simulink model "cycletest_timefeedback"  (R2023a)
settings: Solver=ode1  StartTime=0.0  StopTime=800  FixedStep=0.002  RelTol=1e-3  EnableMultiTasking=on
values from neighbouring files (symbols this model uses):
  cycleGain = 0.2    [simulate_hover.m]    (also in temp.m = 1)
  Jp = 2*Jeq_prop    (= 0.0552224595625)    [setup_lab_hover.m]    (also in simulate_hover.m)
  Jr = 2*Jeq_prop    (= 0.0552224595625)    [setup_lab_hover.m]    (also in simulate_hover.m)
  Jy = 4*Jeq_prop    (= 0.110444919125)    [setup_lab_hover.m]    (also in simulate_hover.m)
  kd = 0.5    [simulate_hover.m]
  Kf = 0.1188    [setup_lab_hover.m]    (also in simulate_hover.m)
  Kt = 0.0036    [setup_lab_hover.m]    (also in simulate_hover.m)
  L = 7.75*0.0254    (= 0.19685)    [setup_lab_hover.m]    (also in simulate_hover.m = 0.1969)
  r = flexSize(no)    [phaseComp.m]    (also in simulate_hover.m = 0.5)
  sigma = 0    [simulate_hover.m]
  skew = 2    [simulate_hover.m]
  V_bias = 12    [setup_lab_hover.m]    (also in simulate_hover.m)
  velMax = 100*60*pi/180    (= 104.71975512)    [simulate_hover.m]
  VMAX_AMP = 24    [setup_lab_hover.m]    (also in simulate_hover.m)
  wcf = 2 * pi * 20    (= 125.663706144)    [setup_lab_hover.m]    (also in simulate_hover.m)
  zetaf = 0.6    [setup_lab_hover.m]    (also in simulate_hover.m)
libraries: simulink_extras x4, dspsrcs4 x1
settings Model: ExtModeTrigDuration=10000  Creator=kille  LastModifiedBy=Jacob
settings SolverCC: AlgebraicLoopSolver=TrustRegion  PositivePriorityOrder=on  AutoInsertRateTranBlk=on
settings DataIOCC: ReturnWorkspaceOutputs=off
settings OptimizationCC: LifeSpan=inf
settings DebuggingCC: UnconnectedInputMsg=warning  UnconnectedOutputMsg=warning  UnconnectedLineMsg=warning  ArithmeticOperatorsInVariantConditions=warning
settings ModelReferenceCC: EnableRefExpFcnMdlSchedulingChecks=on
settings SFSimCC: SimUseLocalCustomCode=off  CustomCodeUndefinedFunction=UseInterfaceOnly
settings RTWCC: Description=QUARC Win64 Target  SystemTargetFile=quarc_win64.tlc  TemplateMakefile=quarc_default_tmf  RTWUseLocalCustomCode=off
settings CodeAppCC: StateflowObjectComments=on
settings STFCustomTargetCC: TargetPreCompLibLocation=C:\PROGRA~3\QUARC\lib\2016a\win64\release  UseToolchainInfoCompliant=off  SystemTargetFile=quarc_win64.tlc
settings GRTTargetCC: TargetPreCompLibLocation=C:\PROGRA~3\QUARC\lib\2016a\win64\release  ParMdlRefBuildCompliant=off  CompOptLevelCompliant=off  CombineOutputUpdateFcns=off  MatFileLogging=off  CPPClassGenCompliant=off  GRTInterface=on  UseToolchainInfoCompliant=off  ExtMode=on  ExtModeMexFile=quarc_comm
settings ConfigComp: CovMetricSettings=dswe

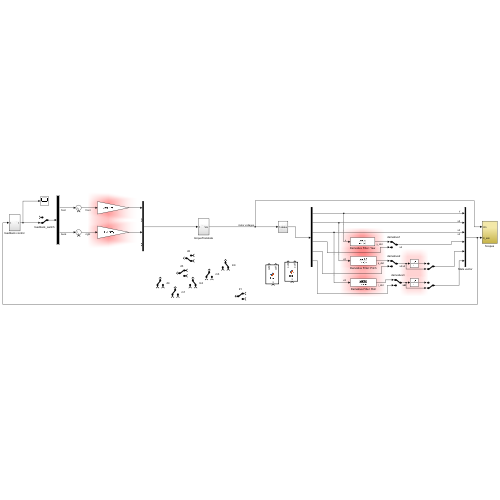
[thumbnail: Simulink's stored preview of the top-level diagram]
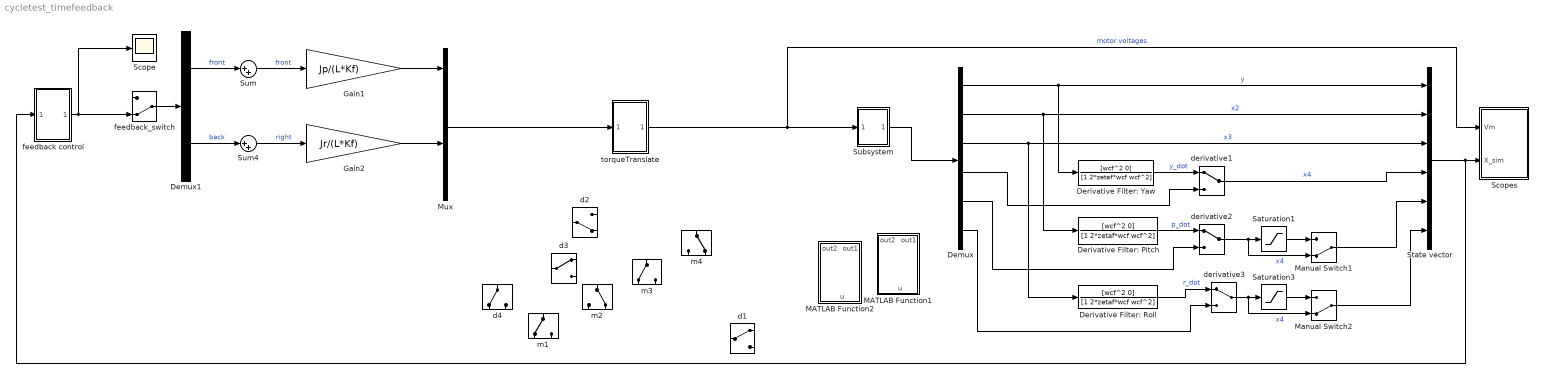
== system cycletest_timefeedback ==
  Demux : Demux  Outputs=6
  Demux1 : Demux  Outputs=2
  Derivative Filter: Pitch : TransferFcn  Numerator=[wcf^2 0]  Denominator=[1 2*zetaf*wcf wcf^2]
  Derivative Filter: Roll : TransferFcn  Numerator=[wcf^2 0]  Denominator=[1 2*zetaf*wcf wcf^2]
  Derivative Filter: Yaw : TransferFcn  Numerator=[wcf^2 0]  Denominator=[1 2*zetaf*wcf wcf^2]
  Gain1 : Gain  Gain=Jp/(L*Kf)
  Gain2 : Gain  Gain=Jr/(L*Kf)
  MATLAB Function1 : MATLAB Function  TreatAsAtomicUnit=on
  MATLAB Function2 : MATLAB Function  TreatAsAtomicUnit=on
  Manual Switch1 : ManualSwitch  CurrentSetting=0
  Manual Switch2 : ManualSwitch  CurrentSetting=0
  Mux : Mux
  Saturation1 : Saturate  UpperLimit=velMax  LowerLimit=-velMax
  Saturation3 : Saturate  UpperLimit=velMax  LowerLimit=-velMax
  Scope : Scope
  Scopes : Subsystem
  State vector : Mux  Inputs=6
  Subsystem : Subsystem
  Sum : Sum  Inputs=|++
  Sum4 : Sum  Inputs=|++
  d1 : ManualSwitch
  d2 : ManualSwitch  CurrentSetting=0
  d3 : ManualSwitch
  d4 : ManualSwitch
  derivative1 : ManualSwitch
  derivative2 : ManualSwitch
  derivative3 : ManualSwitch
  feedback control : Subsystem
  feedback_switch : ManualSwitch  CurrentSetting=0
  m1 : ManualSwitch
  m2 : ManualSwitch  CurrentSetting=0
  m3 : ManualSwitch
  m4 : ManualSwitch  CurrentSetting=0
  torqueTranslate : Subsystem
  wires:
  Demux/1 -> State vector/1, Derivative Filter: Yaw/1  "y"
  torqueTranslate/1(Vm) -> Scopes/1(Vm), Subsystem/1(Input)  "motor voltages"
  Sum4/1 -> Gain2/1  "right"
  Sum/1 -> Gain1/1  "front"
  Mux/1 -> torqueTranslate/1(In1)
  Derivative Filter: Yaw/1 -> derivative1/1  "y_dot"
  Demux/4 -> derivative1/2
  Derivative Filter: Pitch/1 -> derivative2/1  "p_dot"
  Derivative Filter: Roll/1 -> derivative3/1  "r_dot"
  Demux/5 -> derivative2/2
  Demux/6 -> derivative3/2
  derivative1/1 -> State vector/4  "x4"
  derivative2/1 -> Manual Switch1/2, Saturation1/1  "x4"
  Saturation1/1 -> Manual Switch1/1
  derivative3/1 -> Manual Switch2/2, Saturation3/1  "x4"
  Saturation3/1 -> Manual Switch2/1
  Manual Switch1/1 -> State vector/5
  Manual Switch2/1 -> State vector/6
  Demux/3 -> State vector/3, Derivative Filter: Roll/1  "x3"
  Demux/2 -> State vector/2, Derivative Filter: Pitch/1  "x2"
  feedback control/1(Out1) -> Scope/1, feedback_switch/2
  feedback_switch/1 -> Demux1/1
  State vector/1 -> feedback control/1(In1), Scopes/2(X_sim)
  Demux1/1 -> Sum/1  "front"
  Demux1/2 -> Sum4/1  "back"
  Subsystem/1(states) -> Demux/1
  Gain1/1 -> Mux/1
  Gain2/1 -> Mux/3

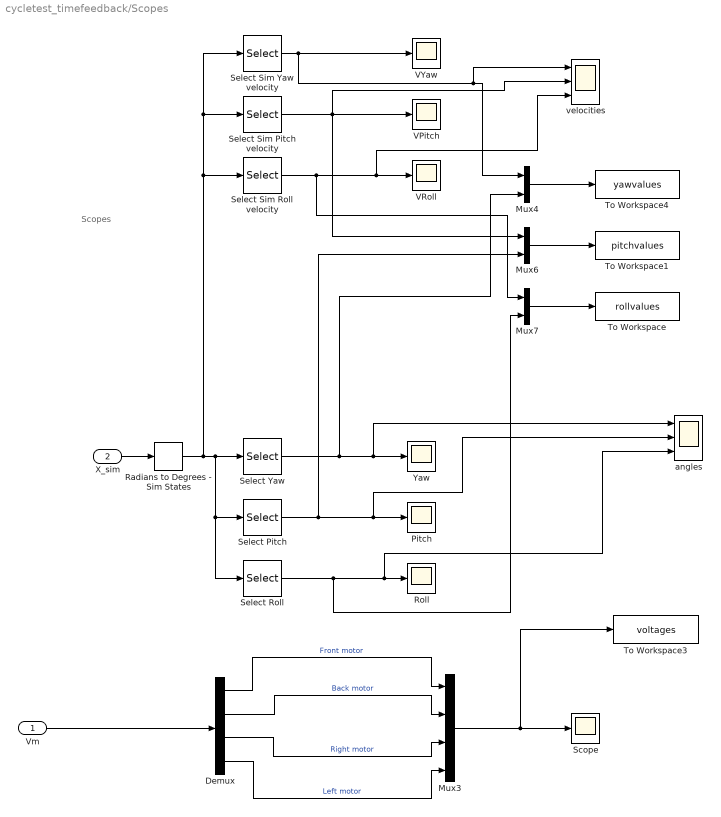
== system cycletest_timefeedback/Scopes ==
  note: Scopes
  Vm : Inport
  X_sim : Inport  Port=2
  Demux : Demux
  Mux3 : Mux
  Mux4 : Mux  Inputs=2
  Mux6 : Mux  Inputs=2
  Mux7 : Mux  Inputs=2
  Pitch : Scope
  Radians to Degrees - Sim States : simulink_extras/Transformations/Radians to Degrees
  Roll : Scope
  Scope : Scope
  Select Pitch : Selector  InputPortWidth=6  IndexOptions=Index vector (dialog)  Indices=2  OutputSizes=1
  Select Roll : Selector  InputPortWidth=6  IndexOptions=Index vector (dialog)  Indices=3  OutputSizes=1
  Select Sim Pitch velocity : Selector  InputPortWidth=6  IndexOptions=Index vector (dialog)  Indices=5  OutputSizes=1
  Select Sim Roll velocity : Selector  InputPortWidth=6  IndexOptions=Index vector (dialog)  Indices=6  OutputSizes=1
  Select Sim Yaw velocity : Selector  InputPortWidth=6  IndexOptions=Index vector (dialog)  Indices=4  OutputSizes=1
  Select Yaw : Selector  InputPortWidth=6  IndexOptions=Index vector (dialog)  Indices=1  OutputSizes=1
  To Workspace : ToWorkspace  VariableName=rollvalues  SampleTime=-1
  To Workspace1 : ToWorkspace  VariableName=pitchvalues  SampleTime=-1
  To Workspace3 : ToWorkspace  VariableName=voltages  SampleTime=-1
  To Workspace4 : ToWorkspace  VariableName=yawvalues  SampleTime=-1
  VPitch : Scope
  VRoll : Scope
  VYaw : Scope
  Yaw : Scope
  angles : Scope  NumInputPorts=3
  velocities : Scope  NumInputPorts=3
  wires:
  Select Roll/1 -> angles/3, Roll/1, Mux7/2
  Radians to Degrees - Sim States/1 -> Select Sim Roll velocity/1, Select Sim Pitch velocity/1, Select Sim Yaw velocity/1, Select Roll/1, Select Pitch/1, Select Yaw/1
  Select Pitch/1 -> angles/2, Pitch/1, Mux6/2
  X_sim/1 -> Radians to Degrees - Sim States/1
  Demux/1 -> Mux3/1  "Front motor"
  Demux/2 -> Mux3/2  "Back motor"
  Demux/3 -> Mux3/3  "Right motor"
  Demux/4 -> Mux3/4  "Left motor"
  Vm/1 -> Demux/1
  Select Sim Yaw velocity/1 -> VYaw/1, velocities/1, Mux4/1
  Select Sim Roll velocity/1 -> velocities/3, VRoll/1, Mux7/1
  Select Sim Pitch velocity/1 -> Mux6/1, velocities/2, VPitch/1
  Mux4/1 -> To Workspace4/1
  Mux6/1 -> To Workspace1/1
  Mux7/1 -> To Workspace/1
  Mux3/1 -> To Workspace3/1, Scope/1
  Select Yaw/1 -> angles/1, Yaw/1, Mux4/2

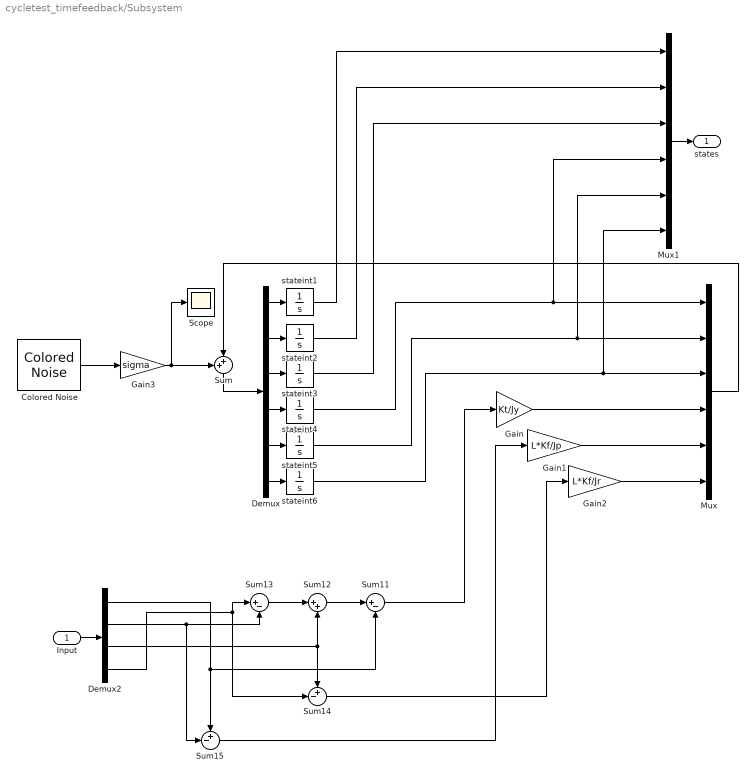
== system cycletest_timefeedback/Subsystem ==
  Input : Inport
  Colored Noise : dspsrcs4/Colored Noise  Color=white  InverseFrequencyPower=1  BoundedOutput=off  NumChannels=6  OutputDataType=double  SamplesPerFrame=1  SampleTime=1  RandomStream=mt19937ar with seed  Seed=67  SimulateUsing=Interpreted execution
  Demux : Demux  Outputs=6
  Demux2 : Demux
  Gain : Gain  Gain=Kt/Jy
  Gain1 : Gain  Gain=L*Kf/Jp
  Gain2 : Gain  Gain=L*Kf/Jr
  Gain3 : Gain  Gain=sigma
  Mux : Mux  Inputs=6
  Mux1 : Mux  Inputs=6
  Scope : Scope
  Sum : Sum  Inputs=++|
  Sum11 : Sum  Inputs=|+-
  Sum12 : Sum  Inputs=|++
  Sum13 : Sum  Inputs=|+-
  Sum14 : Sum  Inputs=+-|
  Sum15 : Sum  Inputs=+-|
  stateint{1,4..6} (4 alike) : Integrator
  stateint2 : Integrator  InitialCondition=0.00010472
  stateint3 : Integrator  InitialCondition=0.00010472
  states : Outport
  wires:
  stateint5/1 -> Mux/2, Mux1/5
  Gain2/1 -> Mux/6
  Gain1/1 -> Mux/5
  stateint6/1 -> Mux/3, Mux1/6
  stateint4/1 -> Mux/1, Mux1/4
  Gain/1 -> Mux/4
  Mux/1 -> Sum/2
  Gain3/1 -> Scope/1, Sum/1
  Demux2/4 -> Sum13/1, Sum14/2
  Demux2/1 -> Sum15/1, Sum11/2
  Demux2/2 -> Sum13/2, Sum15/2
  Sum12/1 -> Sum11/1
  Sum11/1 -> Gain/1
  Demux2/3 -> Sum12/2, Sum14/1
  Sum13/1 -> Sum12/1
  Input/1 -> Demux2/1
  Sum/1 -> Demux/1
  Demux/1 -> stateint1/1
  Demux/2 -> stateint2/1
  Demux/3 -> stateint3/1
  Demux/4 -> stateint4/1
  Demux/5 -> stateint5/1
  Demux/6 -> stateint6/1
  Mux1/1 -> states/1
  stateint1/1 -> Mux1/1
  stateint2/1 -> Mux1/2
  stateint3/1 -> Mux1/3
  Sum15/1 -> Gain1/1
  Sum14/1 -> Gain2/1
  Colored Noise/1 -> Gain3/1

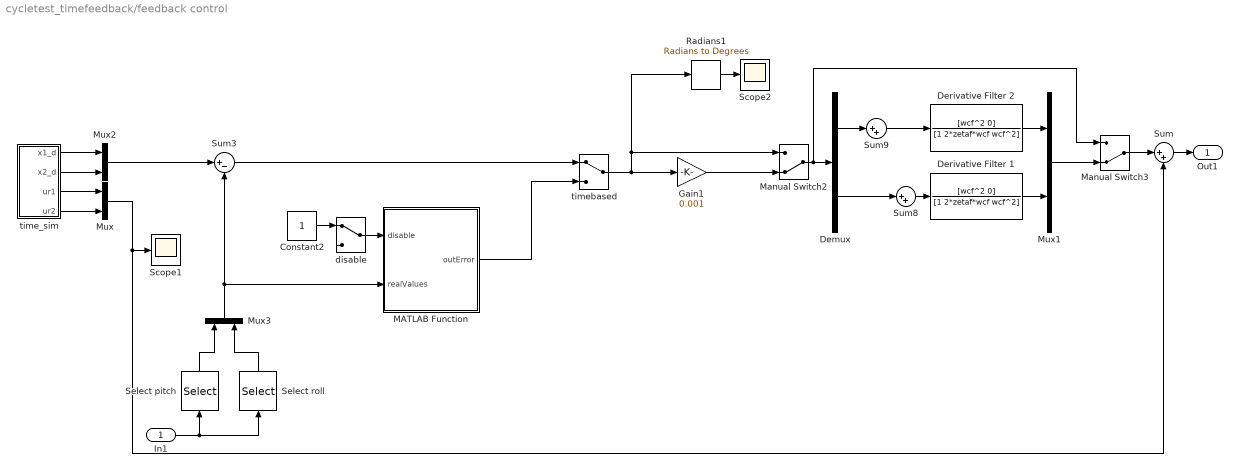
== system cycletest_timefeedback/feedback control ==
  In1 : Inport
  Constant2 : Constant
  Demux : Demux  Outputs=2
  Derivative Filter 1 : TransferFcn  Numerator=[wcf^2 0]  Denominator=[1 2*zetaf*wcf wcf^2]
  Derivative Filter 2 : TransferFcn  Numerator=[wcf^2 0]  Denominator=[1 2*zetaf*wcf wcf^2]
  Gain1 : Gain  Gain=0.001
  MATLAB Function : MATLAB Function  TreatAsAtomicUnit=on
  Manual Switch2 : ManualSwitch  CurrentSetting=0
  Manual Switch3 : ManualSwitch  CurrentSetting=0
  Mux{,1..3} (4 alike) : Mux  Inputs=2
  Radians1 : simulink_extras/Transformations/Radians to Degrees
  Scope1 : Scope
  Scope2 : Scope
  Select pitch : Selector  InputPortWidth=6  IndexOptions=Index vector (dialog)  Indices=2  OutputSizes=1
  Select roll : Selector  InputPortWidth=6  IndexOptions=Index vector (dialog)  Indices=3  OutputSizes=1
  Sum : Sum  Inputs=|++
  Sum3 : Sum  Inputs=|+-
  Sum8 : Sum  Inputs=|++
  Sum9 : Sum  Inputs=|++
  disable : ManualSwitch
  time_sim : Subsystem
  timebased : ManualSwitch
  Out1 : Outport
  wires:
  time_sim/1(x1_d) -> Mux2/1
  time_sim/2(x2_d) -> Mux2/2
  time_sim/4(ur2) -> Mux/2
  time_sim/3(ur1) -> Mux/1
  Sum9/1 -> Derivative Filter 2/1
  Select pitch/1 -> Mux3/1
  Select roll/1 -> Mux3/2
  Sum/1 -> Out1/1
  Sum3/1 -> timebased/1
  Gain1/1 -> Manual Switch2/2
  Mux1/1 -> Manual Switch3/2
  Derivative Filter 2/1 -> Mux1/1
  MATLAB Function/1(outError) -> timebased/2
  Derivative Filter 1/1 -> Mux1/2
  Demux/1 -> Sum9/1
  Mux3/1 -> MATLAB Function/2(realValues), Sum3/2
  Radians1/1 -> Scope2/1
  Manual Switch2/1 -> Manual Switch3/1, Demux/1
  Sum8/1 -> Derivative Filter 1/1
  disable/1 -> MATLAB Function/1(disable)
  In1/1 -> Select roll/1, Select pitch/1
  Mux2/1 -> Sum3/1
  Mux/1 -> Sum/2, Scope1/1
  Constant2/1 -> disable/1
  Demux/2 -> Sum8/1
  Manual Switch3/1 -> Sum/1
  timebased/1 -> Manual Switch2/1, Radians1/1, Gain1/1

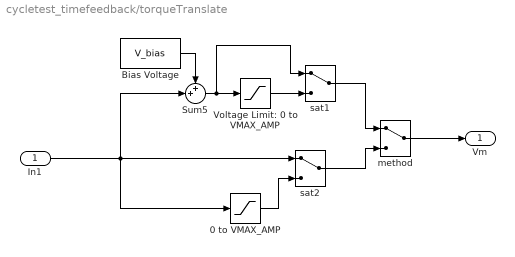
== system cycletest_timefeedback/torqueTranslate ==
  In1 : Inport
  0 to VMAX_AMP : Saturate  UpperLimit=VMAX_AMP  LowerLimit=0
  Bias Voltage : Constant  Value=V_bias
  Sum5 : Sum  Inputs=++|
  Voltage Limit: 0 to VMAX_AMP : Saturate  UpperLimit=VMAX_AMP  LowerLimit=0
  method : ManualSwitch  Tag=swt
  sat1 : ManualSwitch
  sat2 : ManualSwitch
  Vm : Outport
  wires:
  Sum5/1 -> sat1/1, Voltage Limit: 0 to VMAX_AMP/1
  Bias Voltage/1 -> Sum5/1
  Voltage Limit: 0 to VMAX_AMP/1 -> sat1/2
  0 to VMAX_AMP/1 -> sat2/2
  sat1/1 -> method/1
  method/1 -> Vm/1
  sat2/1 -> method/2
  In1/1 -> 0 to VMAX_AMP/1, sat2/1, Sum5/2

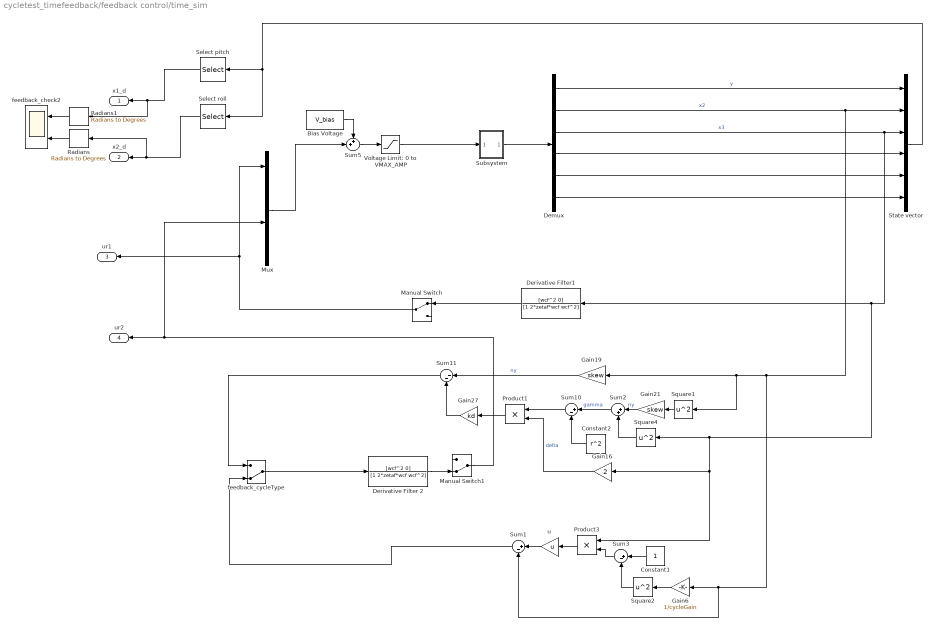
== system cycletest_timefeedback/feedback control/time_sim ==
  Bias Voltage : Constant  Value=V_bias
  Constant1 : Constant
  Constant2 : Constant  Value=r^2
  Demux : Demux  Outputs=6
  Derivative Filter 2 : TransferFcn  Numerator=[wcf^2 0]  Denominator=[1 2*zetaf*wcf wcf^2]
  Derivative Filter1 : TransferFcn  Numerator=[wcf^2 0]  Denominator=[1 2*zetaf*wcf wcf^2]
  Gain16 : Gain  Gain=2
  Gain19 : Gain  Gain=skew
  Gain21 : Gain  Gain=skew
  Gain27 : Gain  Gain=kd
  Gain6 : Gain  Gain=1/cycleGain
  Manual Switch : ManualSwitch
  Manual Switch1 : ManualSwitch  CurrentSetting=0
  Mux : Mux
  Product1 : Product
  Product3 : Product
  Radians : simulink_extras/Transformations/Radians to Degrees
  Radians1 : simulink_extras/Transformations/Radians to Degrees
  Select pitch : Selector  InputPortWidth=6  IndexOptions=Index vector (dialog)  Indices=2  OutputSizes=1
  Select roll : Selector  InputPortWidth=6  IndexOptions=Index vector (dialog)  Indices=3  OutputSizes=1
  Square1 : Math  Operator=square
  Square2 : Math  Operator=square
  Square4 : Math  Operator=square
  State vector : Mux  Inputs=6
  Subsystem : Subsystem
  Sum1 : Sum  Inputs=|+-
  Sum10 : Sum  Inputs=|+-
  Sum11 : Sum  Inputs=|--
  Sum2 : Sum  Inputs=|++
  Sum3 : Sum  Inputs=|+-
  Sum5 : Sum  Inputs=++|
  Voltage Limit: 0 to VMAX_AMP : Saturate  UpperLimit=VMAX_AMP  LowerLimit=0
  feedback_check2 : Scope  NumInputPorts=2
  feedback_cycleType : ManualSwitch  CurrentSetting=0
  u : Gain  Gain=u
  x1_d : Outport
  x2_d : Outport  Port=2
  ur1 : Outport  Port=3
  ur2 : Outport  Port=4
  wires:
  Radians1/1 -> feedback_check2/1
  Radians/1 -> feedback_check2/2
  Bias Voltage/1 -> Sum5/1
  Sum5/1 -> Voltage Limit: 0 to VMAX_AMP/1
  Mux/1 -> Sum5/2
  Select roll/1 -> Radians/1, x2_d/1
  Select pitch/1 -> Radians1/1, x1_d/1
  Demux/4 -> State vector/4
  Demux/6 -> State vector/6
  Subsystem/1(states) -> Demux/1
  Demux/5 -> State vector/5
  Demux/1 -> State vector/1  "y"
  Voltage Limit: 0 to VMAX_AMP/1 -> Subsystem/1(Input)
  State vector/1 -> Select roll/1, Select pitch/1
  Sum1/1 -> feedback_cycleType/2
  Constant1/1 -> Sum3/1
  Gain27/1 -> Sum11/2
  Sum10/1 -> Product1/1
  Product1/1 -> Gain27/1
  feedback_cycleType/1 -> Derivative Filter 2/1
  Derivative Filter 2/1 -> Manual Switch1/2
  Product3/1 -> u/1
  Demux/2 -> State vector/2, Gain6/1, Sum1/2, Square1/1, Gain19/1  "x2"
  Square2/1 -> Sum3/2
  Gain16/1 -> Product1/2  "delta"
  Square1/1 -> Gain21/1
  Sum11/1 -> feedback_cycleType/1
  Sum2/1 -> Sum10/1  "gamma"
  Constant2/1 -> Sum10/2
  Square4/1 -> Sum2/2
  Gain21/1 -> Sum2/1  "ny"
  Derivative Filter1/1 -> Manual Switch/1
  u/1 -> Sum1/1
  Manual Switch1/1 -> Mux/3, ur2/1
  Demux/3 -> Derivative Filter1/1, Product3/1, Gain16/1, Square4/1, State vector/3  "x3"
  Gain19/1 -> Sum11/1  "ny"
  Sum3/1 -> Product3/2
  Manual Switch/1 -> Mux/1, ur1/1
  Gain6/1 -> Square2/1

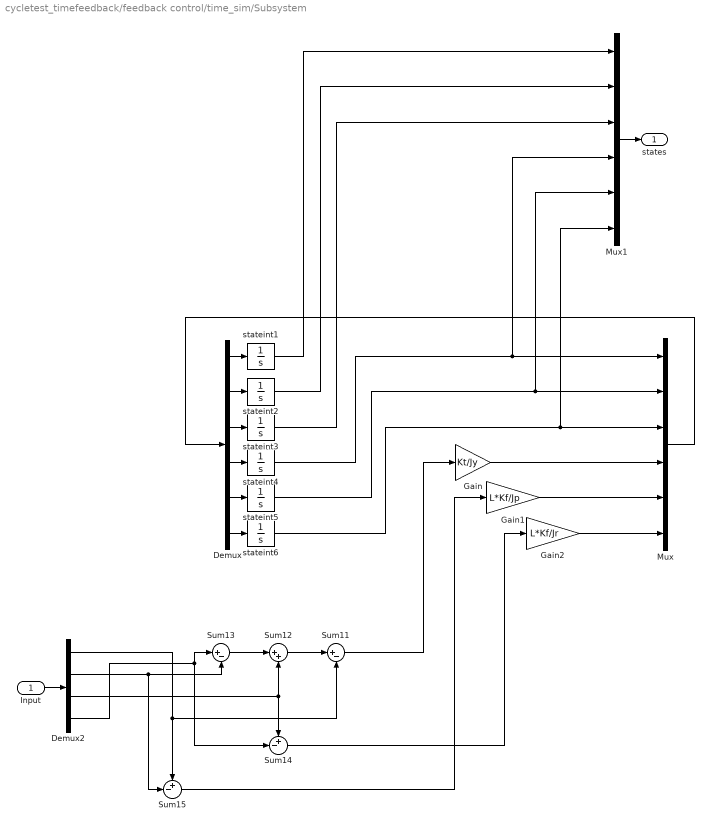
== system cycletest_timefeedback/feedback control/time_sim/Subsystem ==
  Input : Inport
  Demux : Demux  Outputs=6
  Demux2 : Demux
  Gain : Gain  Gain=Kt/Jy
  Gain1 : Gain  Gain=L*Kf/Jp
  Gain2 : Gain  Gain=L*Kf/Jr
  Mux : Mux  Inputs=6
  Mux1 : Mux  Inputs=6
  Sum11 : Sum  Inputs=|+-
  Sum12 : Sum  Inputs=|++
  Sum13 : Sum  Inputs=|+-
  Sum14 : Sum  Inputs=+-|
  Sum15 : Sum  Inputs=+-|
  stateint{1,4..6} (4 alike) : Integrator
  stateint2 : Integrator  InitialCondition=0.00010472
  stateint3 : Integrator  InitialCondition=0.00010472
  states : Outport
  wires:
  stateint5/1 -> Mux/2, Mux1/5
  Gain2/1 -> Mux/6
  Gain1/1 -> Mux/5
  stateint6/1 -> Mux/3, Mux1/6
  stateint4/1 -> Mux/1, Mux1/4
  Gain/1 -> Mux/4
  Demux2/4 -> Sum13/1, Sum14/2
  Demux2/1 -> Sum15/1, Sum11/2
  Demux2/2 -> Sum13/2, Sum15/2
  Sum12/1 -> Sum11/1
  Sum11/1 -> Gain/1
  Demux2/3 -> Sum12/2, Sum14/1
  Sum13/1 -> Sum12/1
  Input/1 -> Demux2/1
  Mux/1 -> Demux/1
  Demux/1 -> stateint1/1
  Demux/2 -> stateint2/1
  Demux/3 -> stateint3/1
  Demux/4 -> stateint4/1
  Demux/5 -> stateint5/1
  Demux/6 -> stateint6/1
  Mux1/1 -> states/1
  stateint1/1 -> Mux1/1
  stateint2/1 -> Mux1/2
  stateint3/1 -> Mux1/3
  Sum15/1 -> Gain1/1
  Sum14/1 -> Gain2/1

== matlab function cycletest_timefeedback/MATLAB Function1 ==
  data: out2 output; u input; out1 output
function [out2, out1] = fcn(u)

if u > 0
    out1 = u;
    out2 = 0;
else
    out1 = 0;
    out2 = -u;
end

== matlab function cycletest_timefeedback/feedback control/MATLAB Function ==
  data: disable input; realValues input; outError output
function outError = approxLimitSimu(disable, realValues)
    outError = [0; 0];
    cyclePoint = [0; 0];
    coder.extrinsic('approxLimit');
    if disable ~= 1
        cyclePoint = approxLimit(realValues);
        outError = cyclePoint-realValues;
    end

== matlab function cycletest_timefeedback/MATLAB Function2 ==
  data: out2 output; u input; out1 output
function [out2, out1] = fcn(u)

if u > 0
    out1 = u;
    out2 = 0;
else
    out1 = 0;
    out2 = -u;
end
